simulink model "ScriptDemo"  (R2022b)
settings: configuration reference "TmVcThermal_Configuration_sub" (kept outside this file)
undefined symbols (not defined in the file or in its folder): aaaa, bbbb, cTmComprCtrl_D_u8HvacFlowTable_db, cTmComprCtrl_D_u8HvacFlowTable_sw, cTmComprCtrl_n_i16ChillCmpIMax, cTmComprCtrl_n_i16ChillCmpIMin, cTmComprCtrl_n_i16ChillCmpIMin666, cTmComprCtrl_n_i16ChillCmpPMax, cTmComprCtrl_n_i16ChillCmpPMin, cTmComprCtrl_n_i16CmpChillCoolRpmKiMax, cTmComprCtrl_n_i16CmpChillCoolRpmKiMin, cTmComprCtrl_n_i16CmpChillCoolRpmKpMax, cTmComprCtrl_n_i16CmpChillCoolRpmKpMin, cTmComprCtrl_n_i16CmpCoolRpmKiMax, cTmComprCtrl_n_i16CmpCoolRpmKiMin, cTmComprCtrl_n_i16CmpCoolRpmKpMax, cTmComprCtrl_n_i16CmpCoolRpmKpMin, cTmComprCtrl_n_i16SM4CmpHeatKiMax, cTmComprCtrl_n_i16SM4CmpHeatKiMin, cTmComprCtrl_n_i16SM4CmpHeatKpMax, cTmComprCtrl_n_i16SM4CmpHeatKpMin, cTmComprCtrl_n_i16SM5CmpHeatKiMax, cTmComprCtrl_n_i16SM5CmpHeatKiMin, cTmComprCtrl_n_i16SM5CmpHeatKpMax, cTmComprCtrl_n_i16SM5CmpHeatKpMin, cTmComprCtrl_n_i16SM6CmpHeatKiMax, cTmComprCtrl_n_i16SM6CmpHeatKiMin, cTmComprCtrl_n_i16SM6CmpHeatKpMax, cTmComprCtrl_n_i16SM6CmpHeatKpMin, cTmComprCtrl_n_u16CmpMaxSpdFanFltLimt, cTmComprCtrl_n_u16CmpMaxSpdLoSidePFltLimt, cTmComprCtrl_n_u16CmpMaxSpdSensorFltLimt, cTmComprCtrl_n_u16CompMinRpm, cTmComprCtrl_n_u16CompRpmIncThres, cTmComprCtrl_t_u16BattCooltFFPeriod, cTmComprCtrl_t_u16BattCooltPIPeriod, cTmComprCtrl_t_u16CmpCoolFFPeriod, cTmComprCtrl_t_u16CmpCoolPIPeriod, cTmComprCtrl_t_u16CoolCmpChillFFPeriod, cTmComprCtrl_t_u16CoolCmpChillPIPeriod, cTmComprCtrl_t_u16SM4CmpHeatFFPeriod, cTmComprCtrl_t_u16SM4CmpHeatPIPeriod, cTmComprCtrl_t_u16SM5CmpHeatFFPeriod, cTmComprCtrl_t_u16SM5CmpHeatPIPeriod, cTmComprCtrl_t_u16SM6CmpHeatFFPeriod, cTmComprCtrl_t_u16SM6CmpHeatPIPeriod, cTmComprCtrl_Te_EvapClearInteg, cTmComprCtrl_Te_i16HpReqTempSaturoffset, cTmComprCtrl_Te_i16SatLpReplaceDiff, cTmComprCtrl_Te_i16SM3BatDiffStartEvapDecOffset, cTmComprCtrl_Te_i16SM3EvapLo, cTmComprCtrl_Te_i16SM3TBatDiffEntEvapDecOffset, cTmComprCtrl_Te_i16SM3TBatDiffEntEvapDecOffsetQuit, cTmComprCtrl_Te_s32ErrCmpChillPIContinueCoolH, cTmComprCtrl_Te_s32ErrCmpChillPIContinueCoolL, cTmComprCtrl_Te_s32ErrCmpPIContinueChillH, cTmComprCtrl_Te_s32ErrCmpPIContinueChillL, cTmComprCtrl_Te_s32ErrCmpPIContinueCoolH, cTmComprCtrl_Te_s32ErrCmpPIContinueCoolL, cTmComprCtrl_Te_s32ErrCmpPIContinueHeatH ... (+398)
libraries: simulink x846, PCMULib x711, simulink_need_slupdate x4
(part 9 of 49)

== system ScriptDemo/Create/createGotoBasedPorts/After ==
  note: createGotoBasedPorts(gcs)
  sTmRefriVlvCtrl_X_s32CEXVPosReqDbgin : Inport  OutDataTypeStr=single
  sTmRefriVlvCtrl_X_s32EEXVPosReqDbgin : Inport  Port=2  OutDataTypeStr=single
  sTmRefriVlvCtrl_X_s32BEXVPosReqDbgin : Inport  Port=3  OutDataTypeStr=single
  yTmRefriVlvCtrl_B_HpcCexvMovEnableDbgin : Inport  Port=4  OutDataTypeStr=boolean
  sTmRefriVlvCtrl_Z_u8CEXVInitStateDbgin : Inport  Port=5  OutDataTypeStr=uint8
  yTmRefriVlvCtrl_B_CexvCalibReqDbgin : Inport  Port=6  OutDataTypeStr=boolean
  yTmRefriVlvCtrl_B_HpcEexvMovEnableDbgin : Inport  Port=7  OutDataTypeStr=boolean
  sTmRefriVlvCtrl_Z_u8EEXVInitStateDbgin : Inport  Port=8  OutDataTypeStr=uint8
  yTmRefriVlvCtrl_B_EexvCalibReqDbgin : Inport  Port=9  OutDataTypeStr=boolean
  yTmRefriVlvCtrl_B_HpcBexvMovEnableDbgin : Inport  Port=10  OutDataTypeStr=boolean
  sTmRefriVlvCtrl_Z_u8BEXVInitStateDbgin : Inport  Port=11  OutDataTypeStr=uint8
  yTmRefriVlvCtrl_B_BexvCalibReqDbgin : Inport  Port=12  OutDataTypeStr=boolean
  sTmRefriVlvCtrl_X_s32SM3BexvMaxPosDbgin : Inport  Port=13  OutDataTypeStr=single
  yTmRefriVlvCtrl_B_EvapBattTLimBexvEnaDbgin : Inport  Port=14  OutDataTypeStr=boolean
  sTmRefriVlvCtrl_D_u8EexvRefriSwitchStDbgin : Inport  Port=15  OutDataTypeStr=uint8
  sTmRefriVlvCtrl_D_u8CexvRefriSwitchStDbgin : Inport  Port=16  OutDataTypeStr=uint8
  sTmRefriVlvCtrl_D_u8BexvRefriSwitchStDbgin : Inport  Port=17  OutDataTypeStr=uint8
  sTmRefriVlvCtrl_X_s32CEXVPosReq : Outport  OutDataTypeStr=single
  sTmRefriVlvCtrl_X_s32EEXVPosReq : Outport  Port=2  OutDataTypeStr=single
  sTmRefriVlvCtrl_X_s32BEXVPosReq : Outport  Port=3  OutDataTypeStr=single
  yTmRefriVlvCtrl_B_HpcCexvMovEnable : Outport  Port=4  OutDataTypeStr=boolean
  sTmRefriVlvCtrl_Z_u8CEXVInitState : Outport  Port=5  OutDataTypeStr=uint8
  yTmRefriVlvCtrl_B_CexvCalibReq : Outport  Port=6  OutDataTypeStr=boolean
  yTmRefriVlvCtrl_B_HpcEexvMovEnable : Outport  Port=7  OutDataTypeStr=boolean
  sTmRefriVlvCtrl_Z_u8EEXVInitState : Outport  Port=8  OutDataTypeStr=uint8
  yTmRefriVlvCtrl_B_EexvCalibReq : Outport  Port=9  OutDataTypeStr=boolean
  yTmRefriVlvCtrl_B_HpcBexvMovEnable : Outport  Port=10  OutDataTypeStr=boolean
  sTmRefriVlvCtrl_Z_u8BEXVInitState : Outport  Port=11  OutDataTypeStr=uint8
  yTmRefriVlvCtrl_B_BexvCalibReq : Outport  Port=12  OutDataTypeStr=boolean
  sTmRefriVlvCtrl_X_s32SM3BexvMaxPos : Outport  Port=13  OutDataTypeStr=single
  yTmRefriVlvCtrl_B_EvapBattTLimBexvEna : Outport  Port=14  OutDataTypeStr=boolean
  sTmRefriVlvCtrl_D_u8EexvRefriSwitchSt : Outport  Port=15  OutDataTypeStr=uint8
  sTmRefriVlvCtrl_D_u8CexvRefriSwitchSt : Outport  Port=16  OutDataTypeStr=uint8
  sTmRefriVlvCtrl_D_u8BexvRefriSwitchSt : Outport  Port=17  OutDataTypeStr=uint8
  wires:
  sTmRefriVlvCtrl_X_s32CEXVPosReqDbgin/1 -> [sTmRefriVlvCtrl_X_s32CEXVPosReqDbgin]
  sTmRefriVlvCtrl_X_s32EEXVPosReqDbgin/1 -> [sTmRefriVlvCtrl_X_s32EEXVPosReqDbgin]
  sTmRefriVlvCtrl_X_s32BEXVPosReqDbgin/1 -> [sTmRefriVlvCtrl_X_s32BEXVPosReqDbgin]
  yTmRefriVlvCtrl_B_HpcCexvMovEnableDbgin/1 -> [yTmRefriVlvCtrl_B_HpcCexvMovEnableDbgin]
  sTmRefriVlvCtrl_Z_u8CEXVInitStateDbgin/1 -> [sTmRefriVlvCtrl_Z_u8CEXVInitStateDbgin]
  yTmRefriVlvCtrl_B_CexvCalibReqDbgin/1 -> [yTmRefriVlvCtrl_B_CexvCalibReqDbgin]
  yTmRefriVlvCtrl_B_HpcEexvMovEnableDbgin/1 -> [yTmRefriVlvCtrl_B_HpcEexvMovEnableDbgin]
  sTmRefriVlvCtrl_Z_u8EEXVInitStateDbgin/1 -> [sTmRefriVlvCtrl_Z_u8EEXVInitStateDbgin]
  yTmRefriVlvCtrl_B_EexvCalibReqDbgin/1 -> [yTmRefriVlvCtrl_B_EexvCalibReqDbgin]
  yTmRefriVlvCtrl_B_HpcBexvMovEnableDbgin/1 -> [yTmRefriVlvCtrl_B_HpcBexvMovEnableDbgin]
  sTmRefriVlvCtrl_Z_u8BEXVInitStateDbgin/1 -> [sTmRefriVlvCtrl_Z_u8BEXVInitStateDbgin]
  yTmRefriVlvCtrl_B_BexvCalibReqDbgin/1 -> [yTmRefriVlvCtrl_B_BexvCalibReqDbgin]
  sTmRefriVlvCtrl_X_s32SM3BexvMaxPosDbgin/1 -> [sTmRefriVlvCtrl_X_s32SM3BexvMaxPosDbgin]
  yTmRefriVlvCtrl_B_EvapBattTLimBexvEnaDbgin/1 -> [yTmRefriVlvCtrl_B_EvapBattTLimBexvEnaDbgin]
  sTmRefriVlvCtrl_D_u8EexvRefriSwitchStDbgin/1 -> [sTmRefriVlvCtrl_D_u8EexvRefriSwitchStDbgin]
  sTmRefriVlvCtrl_D_u8CexvRefriSwitchStDbgin/1 -> [sTmRefriVlvCtrl_D_u8CexvRefriSwitchStDbgin]
  sTmRefriVlvCtrl_D_u8BexvRefriSwitchStDbgin/1 -> [sTmRefriVlvCtrl_D_u8BexvRefriSwitchStDbgin]
  [sTmRefriVlvCtrl_X_s32CEXVPosReq] -> sTmRefriVlvCtrl_X_s32CEXVPosReq/1
  [sTmRefriVlvCtrl_X_s32EEXVPosReq] -> sTmRefriVlvCtrl_X_s32EEXVPosReq/1
  [sTmRefriVlvCtrl_X_s32BEXVPosReq] -> sTmRefriVlvCtrl_X_s32BEXVPosReq/1
  [yTmRefriVlvCtrl_B_HpcCexvMovEnable] -> yTmRefriVlvCtrl_B_HpcCexvMovEnable/1
  [sTmRefriVlvCtrl_Z_u8CEXVInitState] -> sTmRefriVlvCtrl_Z_u8CEXVInitState/1
  [yTmRefriVlvCtrl_B_CexvCalibReq] -> yTmRefriVlvCtrl_B_CexvCalibReq/1
  [yTmRefriVlvCtrl_B_HpcEexvMovEnable] -> yTmRefriVlvCtrl_B_HpcEexvMovEnable/1
  [sTmRefriVlvCtrl_Z_u8EEXVInitState] -> sTmRefriVlvCtrl_Z_u8EEXVInitState/1
  [yTmRefriVlvCtrl_B_EexvCalibReq] -> yTmRefriVlvCtrl_B_EexvCalibReq/1
  [yTmRefriVlvCtrl_B_HpcBexvMovEnable] -> yTmRefriVlvCtrl_B_HpcBexvMovEnable/1
  [sTmRefriVlvCtrl_Z_u8BEXVInitState] -> sTmRefriVlvCtrl_Z_u8BEXVInitState/1
  [yTmRefriVlvCtrl_B_BexvCalibReq] -> yTmRefriVlvCtrl_B_BexvCalibReq/1
  [sTmRefriVlvCtrl_X_s32SM3BexvMaxPos] -> sTmRefriVlvCtrl_X_s32SM3BexvMaxPos/1
  [yTmRefriVlvCtrl_B_EvapBattTLimBexvEna] -> yTmRefriVlvCtrl_B_EvapBattTLimBexvEna/1
  [sTmRefriVlvCtrl_D_u8EexvRefriSwitchSt] -> sTmRefriVlvCtrl_D_u8EexvRefriSwitchSt/1
  [sTmRefriVlvCtrl_D_u8CexvRefriSwitchSt] -> sTmRefriVlvCtrl_D_u8CexvRefriSwitchSt/1
  [sTmRefriVlvCtrl_D_u8BexvRefriSwitchSt] -> sTmRefriVlvCtrl_D_u8BexvRefriSwitchSt/1

== system ScriptDemo/Create/createGotoBasedPorts/Before ==
  sTmRefriVlvCtrl_X_s32CEXVPosReqDbgin : Inport  OutDataTypeStr=single
  sTmRefriVlvCtrl_X_s32EEXVPosReqDbgin : Inport  Port=2  OutDataTypeStr=single
  sTmRefriVlvCtrl_X_s32BEXVPosReqDbgin : Inport  Port=3  OutDataTypeStr=single
  yTmRefriVlvCtrl_B_HpcCexvMovEnableDbgin : Inport  Port=4  OutDataTypeStr=boolean
  sTmRefriVlvCtrl_Z_u8CEXVInitStateDbgin : Inport  Port=5  OutDataTypeStr=uint8
  yTmRefriVlvCtrl_B_CexvCalibReqDbgin : Inport  Port=6  OutDataTypeStr=boolean
  yTmRefriVlvCtrl_B_HpcEexvMovEnableDbgin : Inport  Port=7  OutDataTypeStr=boolean
  sTmRefriVlvCtrl_Z_u8EEXVInitStateDbgin : Inport  Port=8  OutDataTypeStr=uint8
  yTmRefriVlvCtrl_B_EexvCalibReqDbgin : Inport  Port=9  OutDataTypeStr=boolean
  yTmRefriVlvCtrl_B_HpcBexvMovEnableDbgin : Inport  Port=10  OutDataTypeStr=boolean
  sTmRefriVlvCtrl_Z_u8BEXVInitStateDbgin : Inport  Port=11  OutDataTypeStr=uint8
  yTmRefriVlvCtrl_B_BexvCalibReqDbgin : Inport  Port=12  OutDataTypeStr=boolean
  sTmRefriVlvCtrl_X_s32SM3BexvMaxPosDbgin : Inport  Port=13  OutDataTypeStr=single
  yTmRefriVlvCtrl_B_EvapBattTLimBexvEnaDbgin : Inport  Port=14  OutDataTypeStr=boolean
  sTmRefriVlvCtrl_D_u8EexvRefriSwitchStDbgin : Inport  Port=15  OutDataTypeStr=uint8
  sTmRefriVlvCtrl_D_u8CexvRefriSwitchStDbgin : Inport  Port=16  OutDataTypeStr=uint8
  sTmRefriVlvCtrl_D_u8BexvRefriSwitchStDbgin : Inport  Port=17  OutDataTypeStr=uint8
  sTmRefriVlvCtrl_X_s32CEXVPosReq : Outport  OutDataTypeStr=single
  sTmRefriVlvCtrl_X_s32EEXVPosReq : Outport  Port=2  OutDataTypeStr=single
  sTmRefriVlvCtrl_X_s32BEXVPosReq : Outport  Port=3  OutDataTypeStr=single
  yTmRefriVlvCtrl_B_HpcCexvMovEnable : Outport  Port=4  OutDataTypeStr=boolean
  sTmRefriVlvCtrl_Z_u8CEXVInitState : Outport  Port=5  OutDataTypeStr=uint8
  yTmRefriVlvCtrl_B_CexvCalibReq : Outport  Port=6  OutDataTypeStr=boolean
  yTmRefriVlvCtrl_B_HpcEexvMovEnable : Outport  Port=7  OutDataTypeStr=boolean
  sTmRefriVlvCtrl_Z_u8EEXVInitState : Outport  Port=8  OutDataTypeStr=uint8
  yTmRefriVlvCtrl_B_EexvCalibReq : Outport  Port=9  OutDataTypeStr=boolean
  yTmRefriVlvCtrl_B_HpcBexvMovEnable : Outport  Port=10  OutDataTypeStr=boolean
  sTmRefriVlvCtrl_Z_u8BEXVInitState : Outport  Port=11  OutDataTypeStr=uint8
  yTmRefriVlvCtrl_B_BexvCalibReq : Outport  Port=12  OutDataTypeStr=boolean
  sTmRefriVlvCtrl_X_s32SM3BexvMaxPos : Outport  Port=13  OutDataTypeStr=single
  yTmRefriVlvCtrl_B_EvapBattTLimBexvEna : Outport  Port=14  OutDataTypeStr=boolean
  sTmRefriVlvCtrl_D_u8EexvRefriSwitchSt : Outport  Port=15  OutDataTypeStr=uint8
  sTmRefriVlvCtrl_D_u8CexvRefriSwitchSt : Outport  Port=16  OutDataTypeStr=uint8
  sTmRefriVlvCtrl_D_u8BexvRefriSwitchSt : Outport  Port=17  OutDataTypeStr=uint8

== system ScriptDemo/Create/createGotoUseless/After ==
  note: createGotoUseless()
  After : Subsystem
  Ground{,1..8} (9 alike) : Ground
  Terminator{,1..17} (18 alike) : Terminator
  wires:
  [sTmRefriVlvCtrl_Z_u8CEXVInitState] -> After/3(sTmRefriVlvCtrl_Z_u8CEXVInitState)
  After/13(sTmIn_U_s32ElacCmprHvActl) -> [sTmIn_U_s32ElacCmprHvActl]
  [sTmRefriVlvCtrl_Z_u8EEXVInitState] -> After/4(sTmRefriVlvCtrl_Z_u8EEXVInitState)
  After/6(sTmIn_D_u8DCChrgSt) -> [sTmIn_D_u8DCChrgSt]
  ? -> [sTmIn_Te_s32HvBattCooltTReq]
  [sTmDiag_D_u8FanFltSt] -> After/1(sTmDiag_D_u8FanFltSt)
  [sTmSigProces_D_u8BattThermReq] -> After/5(sTmSigProces_D_u8BattThermReq)
  After/15(sTmIn_X_s32CexvPosSts) -> [sTmIn_X_s32CexvPosSts]
  [sTmDiag_D_u8HiSidePFltSt] -> After/2(sTmDiag_D_u8HiSidePFltSt)
  After/14(sTmIn_X_s32BexvPosSts) -> [sTmIn_X_s32BexvPosSts]
  After/3(sTmDiag_D_u8Sov3FltSt) -> [sTmDiag_D_u8Sov3FltSt]
  After/16(sTmSigProces_Te_s32EvapFanReqRamp) -> [sTmSigProces_Te_s32EvapFanReqRamp]
  [sTmSigProces_Te_s32EvapFanFilter] -> After/9(sTmSigProces_Te_s32EvapFanFilter)
  [sTmSigProces_D_u8HvBattCoolgReq] -> After/6(sTmSigProces_D_u8HvBattCoolgReq)
  ? -> [sTmDiag_D_u8BexvFltSt]
  [sTmSigProces_Te_s32CompDischarge] -> After/8(sTmSigProces_Te_s32CompDischarge)
  After/1(TmComprCtrl_100) -> [TmComprCtrl_100]
  After/2(sTmDiag_D_u8CexvFltSt) -> [sTmDiag_D_u8CexvFltSt]
  After/5(sTmDiag_D_u8TeEvapFltSt) -> [sTmDiag_D_u8TeEvapFltSt]
  After/4(sTmDiag_D_u8Sov5FltSt) -> [sTmDiag_D_u8Sov5FltSt]
  [sTmSigProces_D_u8PowerFault] -> After/7(sTmSigProces_D_u8PowerFault)
  After/7(sTmIn_D_u8HeatPump) -> [sTmIn_D_u8HeatPump]
  After/8(sTmIn_D_u8HvActvSts) -> [sTmIn_D_u8HvActvSts]
  After/9(sTmIn_I_s32ElacCmprHvActl) -> [sTmIn_I_s32ElacCmprHvActl]
  After/10(sTmIn_Pw_s32HvCoolgAllwd) -> [sTmIn_Pw_s32HvCoolgAllwd]
  After/11(sTmIn_Te_s32BattHv) -> [sTmIn_Te_s32BattHv]
  After/12(sTmIn_Te_s32HvBattCooltT) -> [sTmIn_Te_s32HvBattCooltT]
  Ground/1 -> [sTmDiag_D_u8FanFltSt]
  Ground1/1 -> [sTmDiag_D_u8HiSidePFltSt]
  Ground2/1 -> [sTmRefriVlvCtrl_Z_u8CEXVInitState]
  Ground3/1 -> [sTmRefriVlvCtrl_Z_u8EEXVInitState]
  Ground4/1 -> [sTmSigProces_D_u8BattThermReq]
  Ground5/1 -> [sTmSigProces_D_u8HvBattCoolgReq]
  Ground6/1 -> [sTmSigProces_D_u8PowerFault]
  Ground7/1 -> [sTmSigProces_Te_s32CompDischarge]
  Ground8/1 -> [sTmSigProces_Te_s32EvapFanFilter]
  [TmComprCtrl_100] -> Terminator/1
  [sTmDiag_D_u8BexvFltSt] -> Terminator1/1
  [sTmIn_Pw_s32HvCoolgAllwd] -> Terminator2/1
  [sTmIn_Te_s32BattHv] -> Terminator3/1
  [sTmIn_Te_s32HvBattCooltT] -> Terminator4/1
  [sTmIn_Te_s32HvBattCooltTReq] -> Terminator5/1
  [sTmIn_U_s32ElacCmprHvActl] -> Terminator6/1
  [sTmIn_X_s32BexvPosSts] -> Terminator7/1
  [sTmIn_X_s32CexvPosSts] -> Terminator8/1
  [sTmSigProces_Te_s32EvapFanReqRamp] -> Terminator9/1
  [sTmDiag_D_u8CexvFltSt] -> Terminator10/1
  [sTmDiag_D_u8Sov3FltSt] -> Terminator11/1
  [sTmDiag_D_u8Sov5FltSt] -> Terminator12/1
  [sTmDiag_D_u8TeEvapFltSt] -> Terminator13/1
  [sTmIn_D_u8DCChrgSt] -> Terminator14/1
  [sTmIn_D_u8HeatPump] -> Terminator15/1
  [sTmIn_D_u8HvActvSts] -> Terminator16/1
  [sTmIn_I_s32ElacCmprHvActl] -> Terminator17/1

== system ScriptDemo/Create/createGotoUseless/Before ==
  After : Subsystem
  wires:
  [sTmRefriVlvCtrl_Z_u8CEXVInitState] -> After/3(sTmRefriVlvCtrl_Z_u8CEXVInitState)
  After/13(sTmIn_U_s32ElacCmprHvActl) -> [sTmIn_U_s32ElacCmprHvActl]
  [sTmRefriVlvCtrl_Z_u8EEXVInitState] -> After/4(sTmRefriVlvCtrl_Z_u8EEXVInitState)
  After/6(sTmIn_D_u8DCChrgSt) -> [sTmIn_D_u8DCChrgSt]
  ? -> [sTmIn_Te_s32HvBattCooltTReq]
  [sTmDiag_D_u8FanFltSt] -> After/1(sTmDiag_D_u8FanFltSt)
  [sTmSigProces_D_u8BattThermReq] -> After/5(sTmSigProces_D_u8BattThermReq)
  After/15(sTmIn_X_s32CexvPosSts) -> [sTmIn_X_s32CexvPosSts]
  [sTmDiag_D_u8HiSidePFltSt] -> After/2(sTmDiag_D_u8HiSidePFltSt)
  After/14(sTmIn_X_s32BexvPosSts) -> [sTmIn_X_s32BexvPosSts]
  After/3(sTmDiag_D_u8Sov3FltSt) -> [sTmDiag_D_u8Sov3FltSt]
  After/16(sTmSigProces_Te_s32EvapFanReqRamp) -> [sTmSigProces_Te_s32EvapFanReqRamp]
  [sTmSigProces_Te_s32EvapFanFilter] -> After/9(sTmSigProces_Te_s32EvapFanFilter)
  [sTmSigProces_D_u8HvBattCoolgReq] -> After/6(sTmSigProces_D_u8HvBattCoolgReq)
  ? -> [sTmDiag_D_u8BexvFltSt]
  [sTmSigProces_Te_s32CompDischarge] -> After/8(sTmSigProces_Te_s32CompDischarge)
  After/1(TmComprCtrl_100) -> [TmComprCtrl_100]
  After/2(sTmDiag_D_u8CexvFltSt) -> [sTmDiag_D_u8CexvFltSt]
  After/5(sTmDiag_D_u8TeEvapFltSt) -> [sTmDiag_D_u8TeEvapFltSt]
  After/4(sTmDiag_D_u8Sov5FltSt) -> [sTmDiag_D_u8Sov5FltSt]
  [sTmSigProces_D_u8PowerFault] -> After/7(sTmSigProces_D_u8PowerFault)
  After/7(sTmIn_D_u8HeatPump) -> [sTmIn_D_u8HeatPump]
  After/8(sTmIn_D_u8HvActvSts) -> [sTmIn_D_u8HvActvSts]
  After/9(sTmIn_I_s32ElacCmprHvActl) -> [sTmIn_I_s32ElacCmprHvActl]
  After/10(sTmIn_Pw_s32HvCoolgAllwd) -> [sTmIn_Pw_s32HvCoolgAllwd]
  After/11(sTmIn_Te_s32BattHv) -> [sTmIn_Te_s32BattHv]
  After/12(sTmIn_Te_s32HvBattCooltT) -> [sTmIn_Te_s32HvBattCooltT]

== system ScriptDemo/Create/createHarness/After ==
  sTmDiag_D_u8CmprDischrgTFltSt : Inport  OutDataTypeStr=uint8
  sTmDiag_D_u8HiSidePFltSt : Inport  Port=2  OutDataTypeStr=uint8
  sTmDiag_D_u8OutrCondOutTFltSt : Inport  Port=3  OutDataTypeStr=uint8
  sTmIn_D_u8HeatPump : Inport  Port=4  OutDataTypeStr=uint8
  sTmDiag_D_u8HiSidePNHPFltSt : Inport  Port=5  OutDataTypeStr=uint8
  Compare To Constant : simulink/Logic and Bit Operations/Compare To Constant  relop=~=  const=0  OutDataTypeStr=boolean
  Compare To Constant1 : simulink/Logic and Bit Operations/Compare To Constant  relop=~=  const=0  OutDataTypeStr=boolean
  Compare To Constant2 : simulink/Logic and Bit Operations/Compare To Constant  relop=~=  const=0  OutDataTypeStr=boolean
  Compare To Constant3 : simulink/Logic and Bit Operations/Compare To Constant  relop===  const=2  OutDataTypeStr=boolean
  Compare To Constant4 : simulink/Logic and Bit Operations/Compare To Constant  relop===  const=2  OutDataTypeStr=boolean
  Compare To Constant5 : simulink/Logic and Bit Operations/Compare To Constant  relop===  const=2  OutDataTypeStr=boolean
  Compare To Constant6 : simulink/Logic and Bit Operations/Compare To Constant  relop===  const=[1 2 3]  OutDataTypeStr=boolean
  Compare To Constant7 : simulink/Logic and Bit Operations/Compare To Constant  relop===  const=1  OutDataTypeStr=boolean
  Constant : Constant  Value=cTmComprCtrl_n_u16CmpMaxSpdSensorFltLimt  OutDataTypeStr=uint16
  Constant1 : Constant  Value=8000  OutDataTypeStr=uint16
  Logical Operator : Logic  Operator=OR  Inputs=4  AllPortsSameDT=off  OutDataTypeStr=boolean
  Logical Operator{1..4} (4 alike) : Logic  AllPortsSameDT=off  OutDataTypeStr=boolean
  Logical Operator5 : Logic  Operator=OR  Inputs=1  AllPortsSameDT=off  OutDataTypeStr=boolean
  Switch : Switch  Criteria=u2 ~= 0  SaturateOnIntegerOverflow=off  InputSameDT=off
  rTmComprCtrl_n_u16CompMaxRpmSensFlt : Outport  OutDataTypeStr=uint16
  xTmComprCtrl_B_CmpSensorFltLimtFlag : Outport  Port=2  OutDataTypeStr=boolean
  wires:
  [sTmDiag_D_u8HiSidePFltSt] -> Compare To Constant/1
  [sTmDiag_D_u8OutrCondOutTFltSt] -> Compare To Constant1/1
  [sTmDiag_D_u8CmprDischrgTFltSt] -> Compare To Constant2/1
  Constant/1 -> Switch/1
  Switch/1 -> [rTmComprCtrl_n_u16CompMaxRpmSensFlt]  "rTmComprCtrl_n_u16CompMaxRpmSensFlt"
  Constant1/1 -> Switch/3
  sTmDiag_D_u8CmprDischrgTFltSt/1 -> [sTmDiag_D_u8CmprDischrgTFltSt]  "sTmDiag_D_u8CmprDischrgTFltSt"
  sTmDiag_D_u8HiSidePFltSt/1 -> [sTmDiag_D_u8HiSidePFltSt]  "sTmDiag_D_u8HiSidePFltSt"
  sTmDiag_D_u8OutrCondOutTFltSt/1 -> [sTmDiag_D_u8OutrCondOutTFltSt]  "sTmDiag_D_u8OutrCondOutTFltSt"
  [rTmComprCtrl_n_u16CompMaxRpmSensFlt] -> rTmComprCtrl_n_u16CompMaxRpmSensFlt/1  "rTmComprCtrl_n_u16CompMaxRpmSensFlt"
  Logical Operator/1 -> [xTmComprCtrl_B_CmpSensorFltLimtFlag]
  [xTmComprCtrl_B_CmpSensorFltLimtFlag] -> xTmComprCtrl_B_CmpSensorFltLimtFlag/1  "xTmComprCtrl_B_CmpSensorFltLimtFlag"
  [xTmComprCtrl_B_CmpSensorFltLimtFlag] -> Switch/2
  [sTmIn_D_u8HeatPump] -> Compare To Constant3/1
  Compare To Constant3/1 -> Logical Operator1/1
  Compare To Constant1/1 -> Logical Operator1/2
  [sTmIn_D_u8HeatPump] -> Compare To Constant4/1
  Compare To Constant4/1 -> Logical Operator2/1
  Compare To Constant2/1 -> Logical Operator2/2
  sTmIn_D_u8HeatPump/1 -> [sTmIn_D_u8HeatPump]  "sTmIn_D_u8HeatPump"
  [sTmIn_D_u8HeatPump] -> Compare To Constant5/1
  Compare To Constant/1 -> Logical Operator3/2
  Compare To Constant5/1 -> Logical Operator3/1
  Compare To Constant6/1 -> Logical Operator5/1
  [sTmIn_D_u8HeatPump] -> Compare To Constant7/1
  [sTmDiag_D_u8HiSidePNHPFltSt] -> Compare To Constant6/1
  Compare To Constant7/1 -> Logical Operator4/1
  Logical Operator1/1 -> Logical Operator/3
  Logical Operator2/1 -> Logical Operator/4
  Logical Operator3/1 -> Logical Operator/2
  Logical Operator4/1 -> Logical Operator/1
  sTmDiag_D_u8HiSidePNHPFltSt/1 -> [sTmDiag_D_u8HiSidePNHPFltSt]  "sTmDiag_D_u8HiSidePNHPFltSt"
  Logical Operator5/1 -> Logical Operator4/2

== system ScriptDemo/Create/createHarness/Before ==
  sTmDiag_D_u8CmprDischrgTFltSt : Inport  OutDataTypeStr=uint8
  sTmDiag_D_u8HiSidePFltSt : Inport  Port=2  OutDataTypeStr=uint8
  sTmDiag_D_u8OutrCondOutTFltSt : Inport  Port=3  OutDataTypeStr=uint8
  sTmIn_D_u8HeatPump : Inport  Port=4  OutDataTypeStr=uint8
  sTmDiag_D_u8HiSidePNHPFltSt : Inport  Port=5  OutDataTypeStr=uint8
  Compare To Constant : simulink/Logic and Bit Operations/Compare To Constant  relop=~=  const=0  OutDataTypeStr=boolean
  Compare To Constant1 : simulink/Logic and Bit Operations/Compare To Constant  relop=~=  const=0  OutDataTypeStr=boolean
  Compare To Constant2 : simulink/Logic and Bit Operations/Compare To Constant  relop=~=  const=0  OutDataTypeStr=boolean
  Compare To Constant3 : simulink/Logic and Bit Operations/Compare To Constant  relop===  const=2  OutDataTypeStr=boolean
  Compare To Constant4 : simulink/Logic and Bit Operations/Compare To Constant  relop===  const=2  OutDataTypeStr=boolean
  Compare To Constant5 : simulink/Logic and Bit Operations/Compare To Constant  relop===  const=2  OutDataTypeStr=boolean
  Compare To Constant6 : simulink/Logic and Bit Operations/Compare To Constant  relop===  const=[1 2 3]  OutDataTypeStr=boolean
  Compare To Constant7 : simulink/Logic and Bit Operations/Compare To Constant  relop===  const=1  OutDataTypeStr=boolean
  Constant : Constant  Value=cTmComprCtrl_n_u16CmpMaxSpdSensorFltLimt  OutDataTypeStr=uint16
  Constant1 : Constant  Value=8000  OutDataTypeStr=uint16
  Logical Operator : Logic  Operator=OR  Inputs=4  AllPortsSameDT=off  OutDataTypeStr=boolean
  Logical Operator{1..4} (4 alike) : Logic  AllPortsSameDT=off  OutDataTypeStr=boolean
  Switch : Switch  Criteria=u2 ~= 0  SaturateOnIntegerOverflow=off  InputSameDT=off
  rTmComprCtrl_n_u16CompMaxRpmSensFlt : Outport  OutDataTypeStr=uint16
  xTmComprCtrl_B_CmpSensorFltLimtFlag : Outport  Port=2  OutDataTypeStr=boolean
  wires:
  [sTmDiag_D_u8HiSidePFltSt] -> Compare To Constant/1
  [sTmDiag_D_u8OutrCondOutTFltSt] -> Compare To Constant1/1
  [sTmDiag_D_u8CmprDischrgTFltSt] -> Compare To Constant2/1
  Constant/1 -> Switch/1
  Switch/1 -> [rTmComprCtrl_n_u16CompMaxRpmSensFlt]  "rTmComprCtrl_n_u16CompMaxRpmSensFlt"
  Constant1/1 -> Switch/3
  sTmDiag_D_u8CmprDischrgTFltSt/1 -> [sTmDiag_D_u8CmprDischrgTFltSt]  "sTmDiag_D_u8CmprDischrgTFltSt"
  sTmDiag_D_u8HiSidePFltSt/1 -> [sTmDiag_D_u8HiSidePFltSt]  "sTmDiag_D_u8HiSidePFltSt"
  sTmDiag_D_u8OutrCondOutTFltSt/1 -> [sTmDiag_D_u8OutrCondOutTFltSt]  "sTmDiag_D_u8OutrCondOutTFltSt"
  [rTmComprCtrl_n_u16CompMaxRpmSensFlt] -> rTmComprCtrl_n_u16CompMaxRpmSensFlt/1  "rTmComprCtrl_n_u16CompMaxRpmSensFlt"
  Logical Operator/1 -> [xTmComprCtrl_B_CmpSensorFltLimtFlag]
  [xTmComprCtrl_B_CmpSensorFltLimtFlag] -> xTmComprCtrl_B_CmpSensorFltLimtFlag/1  "xTmComprCtrl_B_CmpSensorFltLimtFlag"
  [xTmComprCtrl_B_CmpSensorFltLimtFlag] -> Switch/2
  [sTmIn_D_u8HeatPump] -> Compare To Constant3/1
  Compare To Constant3/1 -> Logical Operator1/1
  Compare To Constant1/1 -> Logical Operator1/2
  [sTmIn_D_u8HeatPump] -> Compare To Constant4/1
  Compare To Constant4/1 -> Logical Operator2/1
  Compare To Constant2/1 -> Logical Operator2/2
  sTmIn_D_u8HeatPump/1 -> [sTmIn_D_u8HeatPump]  "sTmIn_D_u8HeatPump"
  [sTmIn_D_u8HeatPump] -> Compare To Constant5/1
  Compare To Constant/1 -> Logical Operator3/2
  Compare To Constant5/1 -> Logical Operator3/1
  Compare To Constant6/1 -> Logical Operator4/2
  [sTmIn_D_u8HeatPump] -> Compare To Constant7/1
  [sTmDiag_D_u8HiSidePNHPFltSt] -> Compare To Constant6/1
  Compare To Constant7/1 -> Logical Operator4/1
  Logical Operator1/1 -> Logical Operator/3
  Logical Operator2/1 -> Logical Operator/4
  Logical Operator3/1 -> Logical Operator/2
  Logical Operator4/1 -> Logical Operator/1
  sTmDiag_D_u8HiSidePNHPFltSt/1 -> [sTmDiag_D_u8HiSidePNHPFltSt]  "sTmDiag_D_u8HiSidePNHPFltSt"

== system ScriptDemo/Create/createHarness/Blue ==
  sTmDiag_D_u8CmprDischrgTFltSt : Inport  OutDataTypeStr=uint8
  sTmDiag_D_u8HiSidePFltSt : Inport  Port=2  OutDataTypeStr=uint8
  sTmDiag_D_u8OutrCondOutTFltSt : Inport  Port=3  OutDataTypeStr=uint8
  sTmIn_D_u8HeatPump : Inport  Port=4  OutDataTypeStr=uint8
  sTmDiag_D_u8HiSidePNHPFltSt : Inport  Port=5  OutDataTypeStr=uint8
  Compare To Constant : simulink/Logic and Bit Operations/Compare To Constant  relop=~=  const=0  OutDataTypeStr=boolean
  Compare To Constant1 : simulink/Logic and Bit Operations/Compare To Constant  relop=~=  const=0  OutDataTypeStr=boolean
  Compare To Constant2 : simulink/Logic and Bit Operations/Compare To Constant  relop=~=  const=0  OutDataTypeStr=boolean
  Compare To Constant3 : simulink/Logic and Bit Operations/Compare To Constant  relop===  const=2  OutDataTypeStr=boolean
  Compare To Constant4 : simulink/Logic and Bit Operations/Compare To Constant  relop===  const=2  OutDataTypeStr=boolean
  Compare To Constant5 : simulink/Logic and Bit Operations/Compare To Constant  relop===  const=2  OutDataTypeStr=boolean
  Compare To Constant6 : simulink/Logic and Bit Operations/Compare To Constant  relop===  const=[1 2 3]  OutDataTypeStr=boolean
  Compare To Constant7 : simulink/Logic and Bit Operations/Compare To Constant  relop===  const=1  OutDataTypeStr=boolean
  Constant : Constant  Value=cTmComprCtrl_n_u16CmpMaxSpdSensorFltLimt  OutDataTypeStr=uint16
  Constant1 : Constant  Value=8000  OutDataTypeStr=uint16
  Logical Operator : Logic  Operator=OR  Inputs=4  AllPortsSameDT=off  OutDataTypeStr=boolean
  Logical Operator{1..4} (4 alike) : Logic  AllPortsSameDT=off  OutDataTypeStr=boolean
  Logical Operator5 : Logic  Operator=OR  Inputs=1  AllPortsSameDT=off  OutDataTypeStr=boolean
  Switch : Switch  Criteria=u2 ~= 0  SaturateOnIntegerOverflow=off  InputSameDT=off
  rTmComprCtrl_n_u16CompMaxRpmSensFlt : Outport  OutDataTypeStr=uint16
  xTmComprCtrl_B_CmpSensorFltLimtFlag : Outport  Port=2  OutDataTypeStr=boolean
  wires:
  [sTmDiag_D_u8HiSidePFltSt] -> Compare To Constant/1
  [sTmDiag_D_u8OutrCondOutTFltSt] -> Compare To Constant1/1
  [sTmDiag_D_u8CmprDischrgTFltSt] -> Compare To Constant2/1
  Constant/1 -> Switch/1
  Switch/1 -> [rTmComprCtrl_n_u16CompMaxRpmSensFlt]  "rTmComprCtrl_n_u16CompMaxRpmSensFlt"
  Constant1/1 -> Switch/3
  sTmDiag_D_u8CmprDischrgTFltSt/1 -> [sTmDiag_D_u8CmprDischrgTFltSt]
  sTmDiag_D_u8HiSidePFltSt/1 -> [sTmDiag_D_u8HiSidePFltSt]
  sTmDiag_D_u8OutrCondOutTFltSt/1 -> [sTmDiag_D_u8OutrCondOutTFltSt]
  [rTmComprCtrl_n_u16CompMaxRpmSensFlt] -> rTmComprCtrl_n_u16CompMaxRpmSensFlt/1
  Logical Operator/1 -> [xTmComprCtrl_B_CmpSensorFltLimtFlag]
  [xTmComprCtrl_B_CmpSensorFltLimtFlag] -> xTmComprCtrl_B_CmpSensorFltLimtFlag/1
  [xTmComprCtrl_B_CmpSensorFltLimtFlag] -> Switch/2
  [sTmIn_D_u8HeatPump] -> Compare To Constant3/1
  Compare To Constant3/1 -> Logical Operator1/1
  Compare To Constant1/1 -> Logical Operator1/2
  [sTmIn_D_u8HeatPump] -> Compare To Constant4/1
  Compare To Constant4/1 -> Logical Operator2/1
  Compare To Constant2/1 -> Logical Operator2/2
  sTmIn_D_u8HeatPump/1 -> [sTmIn_D_u8HeatPump]
  [sTmIn_D_u8HeatPump] -> Compare To Constant5/1
  Compare To Constant/1 -> Logical Operator3/2
  Compare To Constant5/1 -> Logical Operator3/1
  Compare To Constant6/1 -> Logical Operator5/1
  [sTmIn_D_u8HeatPump] -> Compare To Constant7/1
  [sTmDiag_D_u8HiSidePNHPFltSt] -> Compare To Constant6/1
  Compare To Constant7/1 -> Logical Operator4/1
  Logical Operator1/1 -> Logical Operator/3
  Logical Operator2/1 -> Logical Operator/4
  Logical Operator3/1 -> Logical Operator/2
  Logical Operator4/1 -> Logical Operator/1
  sTmDiag_D_u8HiSidePNHPFltSt/1 -> [sTmDiag_D_u8HiSidePNHPFltSt]
  Logical Operator5/1 -> Logical Operator4/2

== system ScriptDemo/Create/createHarness/ID31659_OffCodeState ==
  sTmComprCtrl_D_u32AcOffCode : Inport  OutDataTypeStr=uint32
  sTmComprCtrl_D_u32AcOffCode2 : Inport  Port=2  OutDataTypeStr=uint32
  Bias : Bias  Bias=32  SaturateOnIntegerOverflow=off
  Compare To Constant : simulink/Logic and Bit Operations/Compare To Constant  relop=~=  const=0  OutDataTypeStr=boolean
  Compare To Constant1 : simulink/Logic and Bit Operations/Compare To Constant  relop===  const=0  OutDataTypeStr=boolean
  Data Type Conversion : DataTypeConversion  OutDataTypeStr=uint8  SaturateOnIntegerOverflow=off  RndMeth=Floor
  Data Type Conversion1 : DataTypeConversion  OutDataTypeStr=uint8  SaturateOnIntegerOverflow=off  RndMeth=Floor
  Logical Operator : Logic  Operator=OR  AllPortsSameDT=off  OutDataTypeStr=boolean
  MATLAB Function : MATLAB Function  TreatAsAtomicUnit=on
  MATLAB Function1 : MATLAB Function  TreatAsAtomicUnit=on
  MATLAB Function2 : MATLAB Function  Commented=on  TreatAsAtomicUnit=on
  Switch : Switch  Criteria=u2 ~= 0  SaturateOnIntegerOverflow=off  InputSameDT=off
  Switch1 : Switch  Criteria=u2 ~= 0  SaturateOnIntegerOverflow=off  InputSameDT=off
  Unit Delay : UnitDelay  SampleTime=-1  HasFrameUpgradeWarning=on
  bk : Subsystem  Commented=on
  sTmComprCtrl_D_u8ACOffState : Outport  OutDataTypeStr=uint8
  wires:
  sTmComprCtrl_D_u32AcOffCode/1 -> Compare To Constant/1, MATLAB Function/1(num)  "sTmComprCtrl_D_u32AcOffCode"
  MATLAB Function/1(pos) -> Data Type Conversion/1
  sTmComprCtrl_D_u32AcOffCode2/1 -> Compare To Constant1/1, MATLAB Function1/1(num)  "sTmComprCtrl_D_u32AcOffCode2"
  MATLAB Function1/1(pos) -> Data Type Conversion1/1
  Data Type Conversion/1 -> Switch/1
  Data Type Conversion1/1 -> Bias/1
  Bias/1 -> Switch/3
  Compare To Constant/1 -> Logical Operator/1
  Compare To Constant1/1 -> Logical Operator/2
  Logical Operator/1 -> Switch/2
  Switch/1 -> Switch1/1, Switch1/2
  Switch1/1 -> sTmComprCtrl_D_u8ACOffState/1, Unit Delay/1  "sTmComprCtrl_D_u8ACOffState"
  Unit Delay/1 -> Switch1/3
